simulink model "Simulator_inverse_kinematics_1R2T"  (R2023a)
settings: Solver=VariableStepAuto  StartTime=0.0  StopTime=20.0  RelTol=1e-3
values from neighbouring files (symbols this model uses):
  a1 = A1 - origin    [CDPR_1R2T_test.m]
  a2 = A2 - origin    [CDPR_1R2T_test.m]
  a3 = A3 - origin    [CDPR_1R2T_test.m]
  a4 = A4 - origin    [CDPR_1R2T_test.m]
  b1 = B1 - body_origin    [CDPR_1R2T_test.m]
  b2 = B2 - body_origin    [CDPR_1R2T_test.m]
  r_0 = [0.5 0.5;]'    [CDPR_1R2T_test.m]
  r_end = [0.5 .5]'    [CDPR_1R2T_test.m]
  r_step_time = 5    [CDPR_1R2T_test.m]
  T = 1    [CDPR_1R2T_test.m]
  theta_0 = 0    [CDPR_1R2T_test.m]
  theta_end = 45    [CDPR_1R2T_test.m]
  theta_step_time = 5    [CDPR_1R2T_test.m]
settings Model: Creator=Elias  LastModifiedBy=Elias

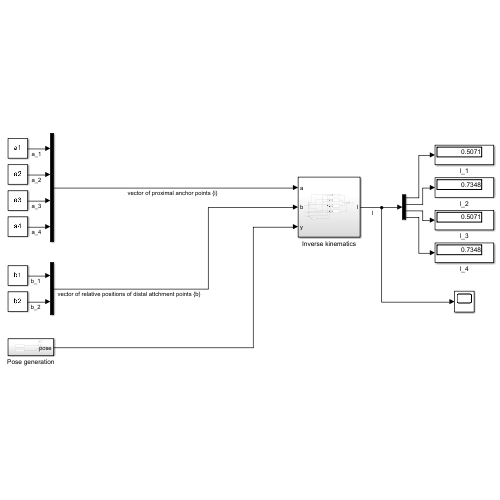
[thumbnail: Simulink's stored preview of the top-level diagram]
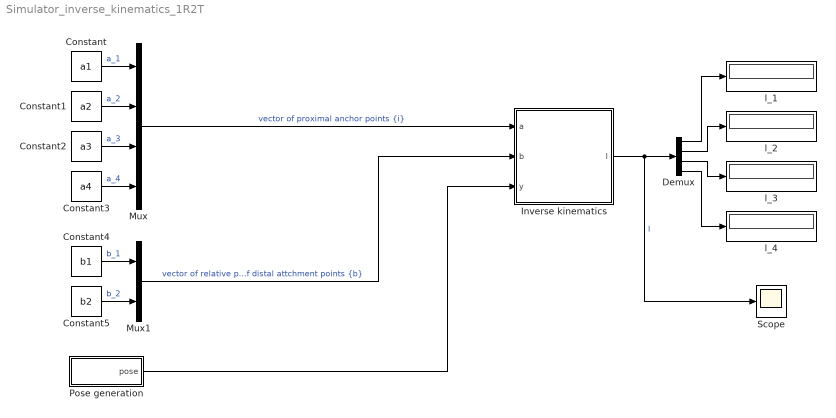
== system Simulator_inverse_kinematics_1R2T ==
  Constant : Constant  Value=a1
  Constant1 : Constant  Value=a2
  Constant2 : Constant  Value=a3
  Constant3 : Constant  Value=a4
  Constant4 : Constant  Value=b1
  Constant5 : Constant  Value=b2
  Demux : Demux
  Inverse kinematics : Subsystem
  Mux : Mux
  Mux1 : Mux  Inputs=2
  Pose generation : Subsystem
  Scope : Scope
  l_{1..4} (4 alike) : Display
  wires:
  Constant/1 -> Mux/1  "a_1"
  Constant1/1 -> Mux/2  "a_2"
  Constant2/1 -> Mux/3  "a_3"
  Constant3/1 -> Mux/4  "a_4"
  Mux/1 -> Inverse kinematics/1(a)  "vector of proximal anchor points {i}"
  Constant4/1 -> Mux1/1  "b_1"
  Constant5/1 -> Mux1/2  "b_2"
  Mux1/1 -> Inverse kinematics/2(b)  "vector of relative positions of distal attchment points {b}"
  Inverse kinematics/1(l) -> Scope/1, Demux/1  "l"
  Demux/1 -> l_1/1
  Demux/2 -> l_2/1
  Demux/3 -> l_3/1
  Demux/4 -> l_4/1
  Pose generation/1(pose) -> Inverse kinematics/3(y)

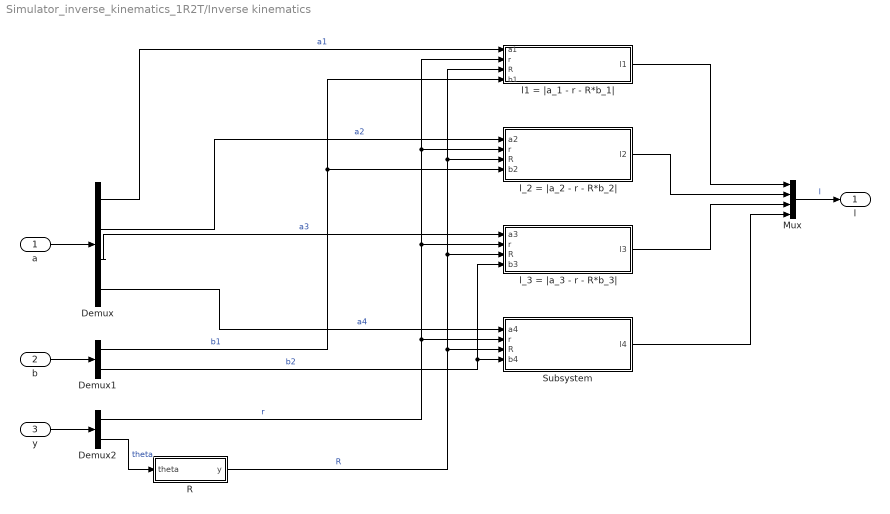
== system Simulator_inverse_kinematics_1R2T/Inverse kinematics ==
  a : Inport
  b : Inport  Port=2
  y : Inport  Port=3
  Demux : Demux
  Demux1 : Demux  Outputs=2
  Demux2 : Demux  Outputs=2
  Mux : Mux
  R : MATLAB Function  TreatAsAtomicUnit=on
  Subsystem : Subsystem
  l1 = |a_1 - r - R*b_1| : Subsystem
  l_2 = |a_2 - r - R*b_2| : Subsystem
  l_3 = |a_3 - r - R*b_3| : Subsystem
  l : Outport
  wires:
  a/1 -> Demux/1
  b/1 -> Demux1/1
  Mux/1 -> l/1  "l"
  y/1 -> Demux2/1
  Demux2/2 -> R/1(theta)  "theta"
  Demux/1 -> l1 = |a_1 - r - R*b_1|/1(a1)  "a1"
  Demux1/1 -> l_2 = |a_2 - r - R*b_2|/4(b2), l1 = |a_1 - r - R*b_1|/4(b1)  "b1"
  Demux2/1 -> l1 = |a_1 - r - R*b_1|/2(r), l_2 = |a_2 - r - R*b_2|/2(r), l_3 = |a_3 - r - R*b_3|/2(r), Subsystem/2(r)  "r"
  R/1(y) -> l1 = |a_1 - r - R*b_1|/3(R), l_2 = |a_2 - r - R*b_2|/3(R), l_3 = |a_3 - r - R*b_3|/3(R), Subsystem/3(R)  "R"
  Demux/2 -> l_2 = |a_2 - r - R*b_2|/1(a2)  "a2"
  Demux/3 -> l_3 = |a_3 - r - R*b_3|/1(a3)  "a3"
  Demux1/2 -> l_3 = |a_3 - r - R*b_3|/4(b3), Subsystem/4(b4)  "b2"
  Demux/4 -> Subsystem/1(a4)  "a4"
  l1 = |a_1 - r - R*b_1|/1(l1) -> Mux/1
  l_2 = |a_2 - r - R*b_2|/1(l2) -> Mux/2
  l_3 = |a_3 - r - R*b_3|/1(l3) -> Mux/3
  Subsystem/1(l4) -> Mux/4

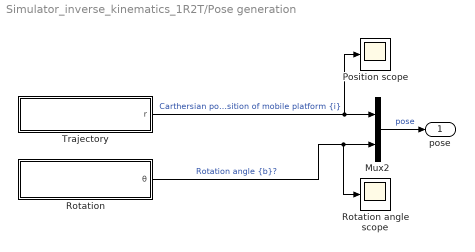
== system Simulator_inverse_kinematics_1R2T/Pose generation ==
  Mux2 : Mux  Inputs=2
  Position scope : Scope
  Rotation : Subsystem
  Rotation angle scope : Scope
  Trajectory : Subsystem
  pose : Outport
  wires:
  Mux2/1 -> pose/1  "pose"
  Trajectory/1(r) -> Position scope/1, Mux2/1  "Carthersian position of mobile platform {i}"
  Rotation/1(θ) -> Rotation angle scope/1, Mux2/2  "Rotation angle {b}?"

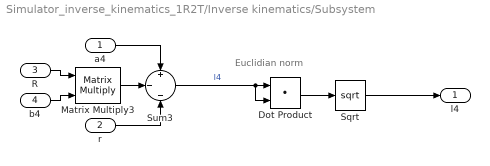
== system Simulator_inverse_kinematics_1R2T/Inverse kinematics/Subsystem ==
  note: Euclidian norm
  a4 : Inport
  r : Inport  Port=2
  R : Inport  Port=3
  b4 : Inport  Port=4
  Dot Product : DotProduct  OutDataTypeStr=Inherit: Inherit via internal rule
  Matrix Multiply3 : Product  Multiplication=Matrix(*)
  Sqrt : Sqrt
  Sum3 : Sum  Inputs=+|-|-
  l4 : Outport
  wires:
  Matrix Multiply3/1 -> Sum3/2
  R/1 -> Matrix Multiply3/1
  a4/1 -> Sum3/1
  r/1 -> Sum3/3
  b4/1 -> Matrix Multiply3/2
  Sum3/1 -> Dot Product/2, Dot Product/1  "l4"
  Sqrt/1 -> l4/1
  Dot Product/1 -> Sqrt/1

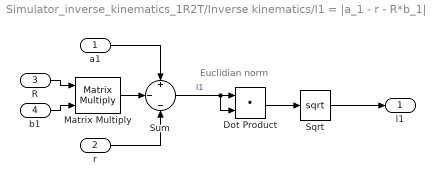
== system Simulator_inverse_kinematics_1R2T/Inverse kinematics/l1 = |a_1 - r - R*b_1| ==
  note: Euclidian norm
  a1 : Inport
  r : Inport  Port=2
  R : Inport  Port=3
  b1 : Inport  Port=4
  Dot Product : DotProduct  OutDataTypeStr=Inherit: Inherit via internal rule
  Matrix Multiply : Product  Multiplication=Matrix(*)
  Sqrt : Sqrt
  Sum : Sum  Inputs=+|-|-
  l1 : Outport
  wires:
  Matrix Multiply/1 -> Sum/2
  a1/1 -> Sum/1
  b1/1 -> Matrix Multiply/2
  r/1 -> Sum/3
  Sum/1 -> Dot Product/2, Dot Product/1  "l1"
  R/1 -> Matrix Multiply/1
  Dot Product/1 -> Sqrt/1
  Sqrt/1 -> l1/1

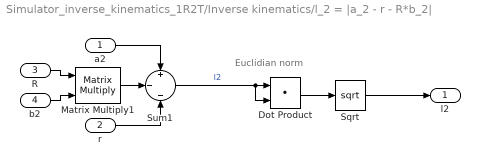
== system Simulator_inverse_kinematics_1R2T/Inverse kinematics/l_2 = |a_2 - r - R*b_2| ==
  note: Euclidian norm
  a2 : Inport
  r : Inport  Port=2
  R : Inport  Port=3
  b2 : Inport  Port=4
  Dot Product : DotProduct  OutDataTypeStr=Inherit: Inherit via internal rule
  Matrix Multiply1 : Product  Multiplication=Matrix(*)
  Sqrt : Sqrt
  Sum1 : Sum  Inputs=+|-|-
  l2 : Outport
  wires:
  Matrix Multiply1/1 -> Sum1/2
  R/1 -> Matrix Multiply1/1
  a2/1 -> Sum1/1
  r/1 -> Sum1/3
  Sum1/1 -> Dot Product/2, Dot Product/1  "l2"
  b2/1 -> Matrix Multiply1/2
  Sqrt/1 -> l2/1
  Dot Product/1 -> Sqrt/1

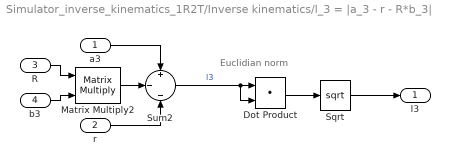
== system Simulator_inverse_kinematics_1R2T/Inverse kinematics/l_3 = |a_3 - r - R*b_3| ==
  note: Euclidian norm
  a3 : Inport
  r : Inport  Port=2
  R : Inport  Port=3
  b3 : Inport  Port=4
  Dot Product : DotProduct  OutDataTypeStr=Inherit: Inherit via internal rule
  Matrix Multiply2 : Product  Multiplication=Matrix(*)
  Sqrt : Sqrt
  Sum2 : Sum  Inputs=+|-|-
  l3 : Outport
  wires:
  a3/1 -> Sum2/1
  R/1 -> Matrix Multiply2/1
  r/1 -> Sum2/3
  b3/1 -> Matrix Multiply2/2
  Matrix Multiply2/1 -> Sum2/2
  Sum2/1 -> Dot Product/2, Dot Product/1  "l3"
  Sqrt/1 -> l3/1
  Dot Product/1 -> Sqrt/1

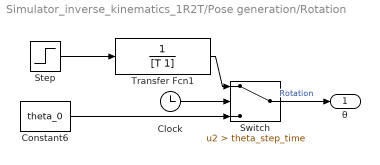
== system Simulator_inverse_kinematics_1R2T/Pose generation/Rotation ==
  Clock : Clock
  Constant6 : Constant  Value=theta_0
  Step : Step  Time=theta_step_time  Before=theta_0  After=theta_end  SampleTime=0
  Switch : Switch  Criteria=u2 > Threshold  Threshold=theta_step_time  SaturateOnIntegerOverflow=off  InputSameDT=off
  Transfer Fcn1 : TransferFcn  Denominator=[T 1]
  θ : Outport
  wires:
  Clock/1 -> Switch/2
  Transfer Fcn1/1 -> Switch/1
  Constant6/1 -> Switch/3
  Step/1 -> Transfer Fcn1/1
  Switch/1 -> θ/1  "Rotation"

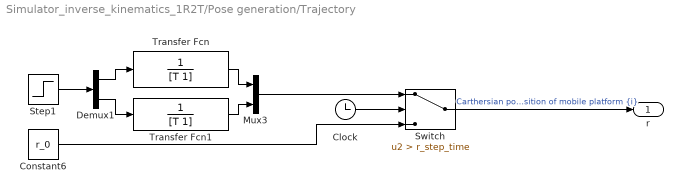
== system Simulator_inverse_kinematics_1R2T/Pose generation/Trajectory ==
  Clock : Clock
  Constant6 : Constant  Value=r_0
  Demux1 : Demux  Outputs=2
  Mux3 : Mux  Inputs=2
  Step1 : Step  Time=r_step_time  Before=r_0  After=r_end  SampleTime=0
  Switch : Switch  Criteria=u2 > Threshold  Threshold=r_step_time  SaturateOnIntegerOverflow=off  InputSameDT=off
  Transfer Fcn : TransferFcn  Denominator=[T 1]
  Transfer Fcn1 : TransferFcn  Denominator=[T 1]
  r : Outport
  wires:
  Demux1/2 -> Transfer Fcn1/1
  Transfer Fcn1/1 -> Mux3/2
  Step1/1 -> Demux1/1
  Clock/1 -> Switch/2
  Demux1/1 -> Transfer Fcn/1
  Transfer Fcn/1 -> Mux3/1
  Constant6/1 -> Switch/3
  Mux3/1 -> Switch/1
  Switch/1 -> r/1  "Carthersian position of mobile platform {i}"

== matlab function Simulator_inverse_kinematics_1R2T/Inverse kinematics/R ==
  data: theta input; y output
function y = R(theta)
% 2D rotation matrix about the 'z'-axis in degrees
y = [cosd(theta) -sind(theta); sind(theta) cosd(theta)];
